simulink model "Microwave"  (R2020a)
settings: Solver=VariableStepAuto  StartTime=0.0  StopTime=500  RelTol=1e-3
settings Model: EnablePacing=on  PacingRate=3  Creator=vivek vivian  LastModifiedBy=vivek vivian

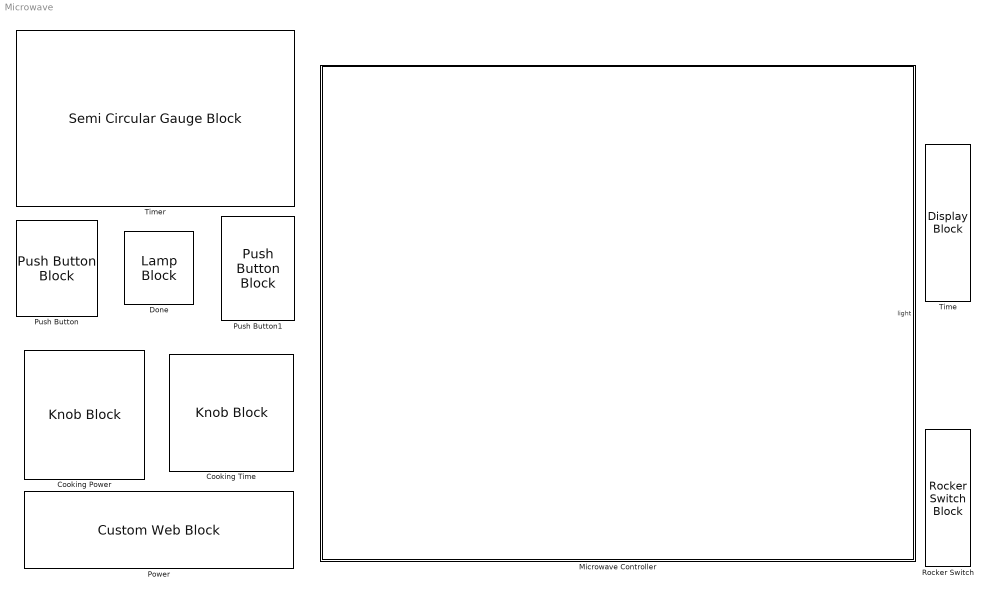
== system Microwave ==
  Cooking Power : KnobBlock  ScaleMax=800
  Cooking Time : KnobBlock  ScaleMax=1000
  Done : LampBlock
  Microwave Controller : Subsystem
  Power : CustomWebBlock  ShowInitialText=on  Configuration="{\"components\":[{\"name\":\"LinearScaleComponent\",\"settings\":{\"bounds\":{\"max\":800,\"min\":0,\"tickInterval\":\"auto\"},\"labelColor\":[250,245,199],\"labelFont\":{\"font\":\"Arial\",\"fontSize\":12},\"labelTransparency\":1,\"needleImage\":{\"size\":[21,75],\"src\":\"data:image\\/svg+xml;base64,PHN2ZyB4bWxucz0iaHR0cDovL3d3dy53My5vcmcvMjAwMC9zdmciIHhtbG5zOnhsaW5rPSJodHRwOi8vd3d3LnczLm9yZy8xOTk5L3hsaW5rIiB2aWV3Qm94PSIwIDAgMjEgNzUiPjxkZWZzPjxzdHlsZT4uY2xzLTF7ZmlsbDpub25lO30uY2xzLTJ7aXNvbGF0aW9uOmlzb2xhdGU7fS5jbHMtM3tjbGlwLXBhdGg6dXJsKCNjbGlwLXBhdGgpO30uY2xzLTR7b3BhY2l0eTowLjM7bWl4LWJsZW5kLW1vZGU6bXVsdGlwbHk7fS5jbHMtNXtmaWxsOiNlYjI2Mjk7fTwvc3R5bGU+PGNsaXBQYXRoIGlkPSJjbGlwLXBhdGgiIHRyYW5zZm9y ...(+1928 chars)\",\"srcOrientation\":\"horizontal\"},\"needleOffset\":[0,0.01094391244870041],\"needleSize\":{\"height\":0.7589285714285714,\"width\":0.11960078534031414},\"position\":[0.069580078125,0.019997667910447763,0.9640858208955224,0.799560546875],\"scaleColorSize\":0.24,\"scaleColors\":[],\"scaleColorsSize\":0.2,\"tickColor\":[250,245,200],\"tickTransparency\":1,\"valueBarColor\":[23,89,176],\"valueBarSize\":0.23,\"valueBarTransparency\":1}},{\"name\":\"BackgroundImageComponent\",\"settings\":{\"image\":{\"size\":[380,101],\"src\":\"data:image\\/svg+xml;base64,PHN2ZyB4bWxucz0iaHR0cDovL3d3dy53My5vcmcvMjAwMC9zdmciIHhtbG5zOnhsaW5rPSJodHRwOi8vd3d3LnczLm9yZy8xOTk5L3hsaW5rIiB2aWV3Qm94PSIwIDAgMzgwIDEwMSI+PGRlZnM+PHN0eWxlPi5jbHMtMXtmaWxsOnVybCgjbGluZWFyLWdyYWRpZW50KTt9LmNscy0ye2ZpbGw6dXJsKCNsaW5lYXItZ3JhZGllbnQtMik7fS5jbHMtM3tmaWxsOnVybCgjbGluZWFyLWdyYWRpZW50LTMpO308L3N0eWxlPjxsaW5lYXJHcmFkaWVudCBpZD0ibGluZWFyLWdyYWRpZW50IiB5MT0iNTAuNSIgeDI9IjM5OS4yOCIgeTI9IjUw ...(+2216 chars)\",\"srcOrientation\":\"horizontal\"},\"position\":[0,0,1,1],\"scaleMode\":\"0\"}}],\"settings\":{\"BindingType\":\"signal\",\"fixedAspectRatio\":\"on\",\"orientation\":\"horizontal\"},\"type\":\"LinearGauge\"}"
  Push Button : PushButtonBlock  ButtonText=START
  Push Button1 : PushButtonBlock  ButtonText=STOP
  Rocker Switch : RockerSwitchBlock
      settings: Values={{'OPEN', 'CLOSE'}, [0 1]}
  Time : DisplayBlock  LabelPosition=Hide  Format=short  Transparency=1
  Timer : SemiCircularGaugeBlock  ScaleMax=1000

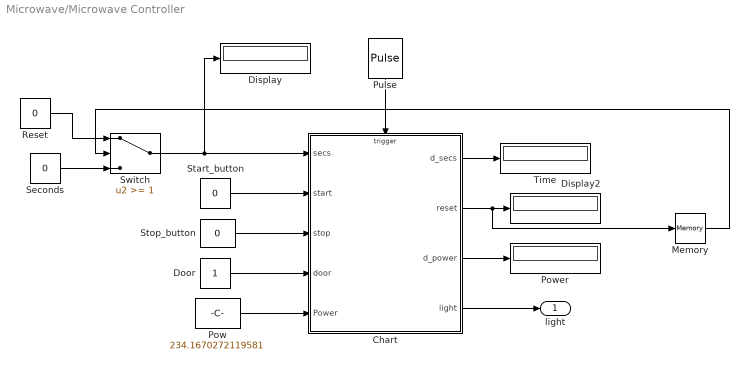
== system Microwave/Microwave Controller ==
  Chart : Stateflow chart  TreatAsAtomicUnit=on
  Display : Display
  Display2 : Display
  Door : Constant
  Memory : Memory  InitialCondition=1
  Pow : Constant  Value=234.1670272119581  OutDataTypeStr=uint32
  Power : Display
  Pulse : DiscretePulseGenerator  PulseType=Time based  Period=1  PulseWidth=5
  Reset : Constant  Value=0  OutDataTypeStr=uint32
  Seconds : Constant  Value=0  OutDataTypeStr=uint32
  Start_button : Constant  Value=0
  Stop_button : Constant  Value=0
  Switch : Switch  Threshold=1
  Time : Display
  light : Outport
  wires:
  Door/1 -> Chart/4(door)
  Chart/3(d_power) -> Power/1
  Chart/2(reset) -> Memory/1, Display2/1
  Start_button/1 -> Chart/2(start)
  Chart/1(d_secs) -> Time/1
  Stop_button/1 -> Chart/3(stop)
  Pow/1 -> Chart/5(Power)
  Pulse/1 -> Chart/Trigger
  Chart/4(light) -> light/1
  Seconds/1 -> Switch/3
  Memory/1 -> Switch/2
  Reset/1 -> Switch/1
  Switch/1 -> Chart/1(secs), Display/1

== stateflow chart Microwave/Microwave Controller/Chart ==
  settings: executeAtInitialization=1
  state Microwave
    en:d_secs=0;sec=0;d_power=0;light=0;reset=0;
    du:count=secs;count_in=secs;d_secs=secs;
    d_power=Power;
  state stop
    en:en=0;
    du:d_secs=count_in;light=0;
    d_power=Power;
    on TIC:Inactive()
    if en==1
    reset=0;
    end;
    ex:sec=0;
  state Cooking
    du:d_secs=count_in;count=secs;
    d_power=Power;
    on TIC:count_in=count_in-1;
  state Check
    en:count_in=secs
    count=secs;
  stop -> Microwave [order 3] : [reset==0]
  stop -> Microwave [order 2] : [stop==1||count==0]
  (default) -> Microwave
  Cooking -> stop [order 4] : [count_in==0]{reset=1;light=1}
  Cooking -> stop [order 1] : [door==0]{reset=1}
  Microwave -> Cooking : [start==1&&door==1]
  Cooking -> stop [order 2] : [stop==1]{reset=1}
  Cooking -> Check [order 3] : [count>secs||count<secs]
  Check -> Cooking : [count_in>=0]
  stop -> Cooking [order 1] : [start==1&&door==1]{reset=0}
  data: d_secs output uint32; secs input uint32; count local uint32; start input; stop input; door input; count_in local uint32; reset output; sec local; en local; Power input; d_power output uint32; light output
  events: TIC input RISING_EDGE_EVENT
  function Inactive:
    | function Inactive
    | sec = sec+1;
    | if sec == 300
    |     en=1;
    | end
